simulink model "PBMAmodel"  (R2014a)
settings: Solver=FixedStepDiscrete  StartTime=0.0  StopTime=8000  RelTol=1e-3
undefined symbols (not defined in the file): pbma_model1
libraries: identextras x30, simulink x16
(part 3 of 3)

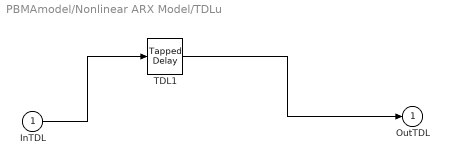
== system PBMAmodel/Nonlinear ARX Model/TDLu ==
  InTDL : Inport
  TDL1 : simulink/Discrete/Tapped Delay  vinit=[0;0]  samptime=1  NumDelays=2  DelayOrder=Newest  includeCurrent=off
  OutTDL : Outport
  wires:
  InTDL/1 -> TDL1/1
  TDL1/1 -> OutTDL/1

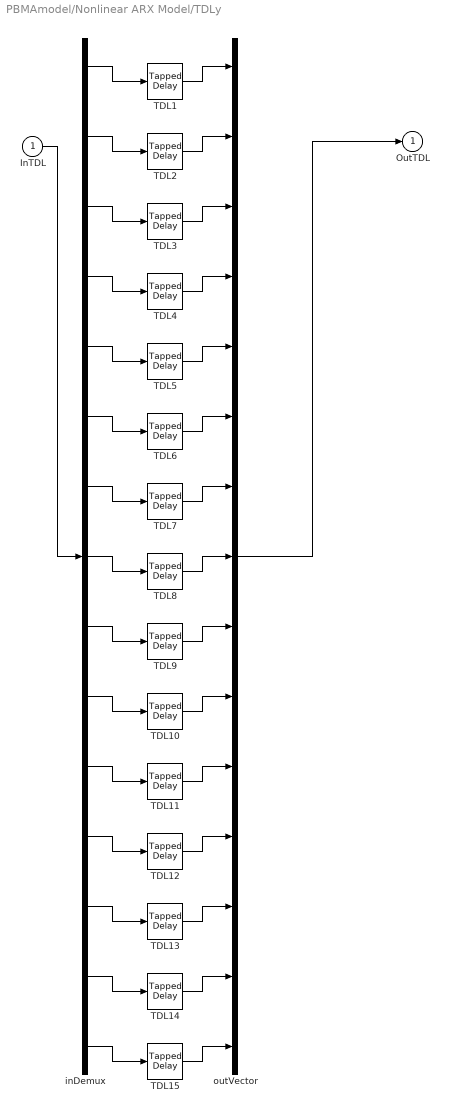
== system PBMAmodel/Nonlinear ARX Model/TDLy ==
  InTDL : Inport
  TDL{1..15} (15 alike) : simulink/Discrete/Tapped Delay  vinit=[0;0]  samptime=1  NumDelays=2  DelayOrder=Newest  includeCurrent=off
  inDemux : Demux  Outputs=15
  outVector : Concatenate  NumInputs=15
  OutTDL : Outport
  wires:
  InTDL/1 -> inDemux/1
  outVector/1 -> OutTDL/1
  inDemux/1 -> TDL1/1
  TDL1/1 -> outVector/1
  inDemux/2 -> TDL2/1
  TDL2/1 -> outVector/2
  inDemux/3 -> TDL3/1
  TDL3/1 -> outVector/3
  inDemux/4 -> TDL4/1
  TDL4/1 -> outVector/4
  inDemux/5 -> TDL5/1
  TDL5/1 -> outVector/5
  inDemux/6 -> TDL6/1
  TDL6/1 -> outVector/6
  inDemux/7 -> TDL7/1
  TDL7/1 -> outVector/7
  inDemux/8 -> TDL8/1
  TDL8/1 -> outVector/8
  inDemux/9 -> TDL9/1
  TDL9/1 -> outVector/9
  inDemux/10 -> TDL10/1
  TDL10/1 -> outVector/10
  inDemux/11 -> TDL11/1
  TDL11/1 -> outVector/11
  inDemux/12 -> TDL12/1
  TDL12/1 -> outVector/12
  inDemux/13 -> TDL13/1
  TDL13/1 -> outVector/13
  inDemux/14 -> TDL14/1
  TDL14/1 -> outVector/14
  inDemux/15 -> TDL15/1
  TDL15/1 -> outVector/15
